simulink model "untitled"  (R2018a)
settings: Solver=VariableStepAuto  StartTime=0.0  StopTime=10.0  RelTol=1e-3
settings Model: Creator=25593  LastModifiedBy=25593

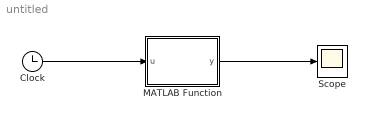
== system untitled ==
  Clock : Clock
  MATLAB Function : MATLAB Function  TreatAsAtomicUnit=on
  Scope : Scope
  wires:
  MATLAB Function/1(y) -> Scope/1
  Clock/1 -> MATLAB Function/1(u)

== matlab function untitled/MATLAB Function ==
  data: u input; y output
function y = fcn(u)
y = u;
